simulink model "dynamic_model"  (R2016b)
settings: Solver=ode3  StartTime=0.0  StopTime=inf  FixedStep=0.001  MaxStep=0.004  RelTol=1e-3
undefined symbols (not defined in the file): deg, rad, s
libraries: simulink x6, aerolibconvert2 x3, aerolibobsolete x1, aerolibtransform2 x1, aerolibatmos2 x1, aerolibnav x1, aerolibanimutils x1
settings Model: Creator=ADAM  LastModifiedBy=consti
settings SolverCC: ExtrapolationOrder=1
settings DataIOCC: MaxDataPoints=1  SaveFormat=Structure  SignalLoggingSaveFormat=ModelDataLogs  SaveOutput=off  SignalLogging=off  DSMLogging=off  SaveTime=off  OutputSaveName=model_out  SignalLoggingName=model_out
settings OptimizationCC: ExpressionDepthLimit=2147483647  LifeSpan=inf  SimCompilerOptimization=on
settings DebuggingCC: UnderspecifiedInitializationDetection=Classic  MergeDetectMultiDrivingBlocksExec=none  SolverPrmCheckMsg=warning  InheritedTsInSrcMsg=none  MultiTaskDSMMsg=warning  MultiTaskCondExecSysMsg=none  UnconnectedInputMsg=none  UnconnectedOutputMsg=none  UnconnectedLineMsg=none  StateNameClashWarn=warning  SFUnexpectedBacktrackingDiag=warning  SFNoUnconditionalDefaultTransitionDiag=warning  SFExecutionAtInitializationDiag=none
settings HardwareCC: ProdBitPerPointer=32  ProdBitPerSizeT=32  ProdBitPerPtrDiffT=32  ProdLargestAtomicFloat=None  ProdWordSize=32  ProdHWDeviceType=Generic->32-bit x86 compatible
settings ModelReferenceCC: ModelReferenceNumInstancesAllowed=Single  PropagateSignalLabelsOutOfModel=off
settings CodeAppCC: MaxIdLength=95
settings GRTTargetCC: TargetLangStandard=C89/C90 (ANSI)  GeneratePreprocessorConditionals=Disable all
settings ConfigComp: CovMetricSettings=dw  CovHtmlReporting=on  CovSaveCumulativeToWorkspaceVar=on  CovSaveSingleToWorkspaceVar=on  CovExternalEMLEnable=off  CovSFcnEnable=off

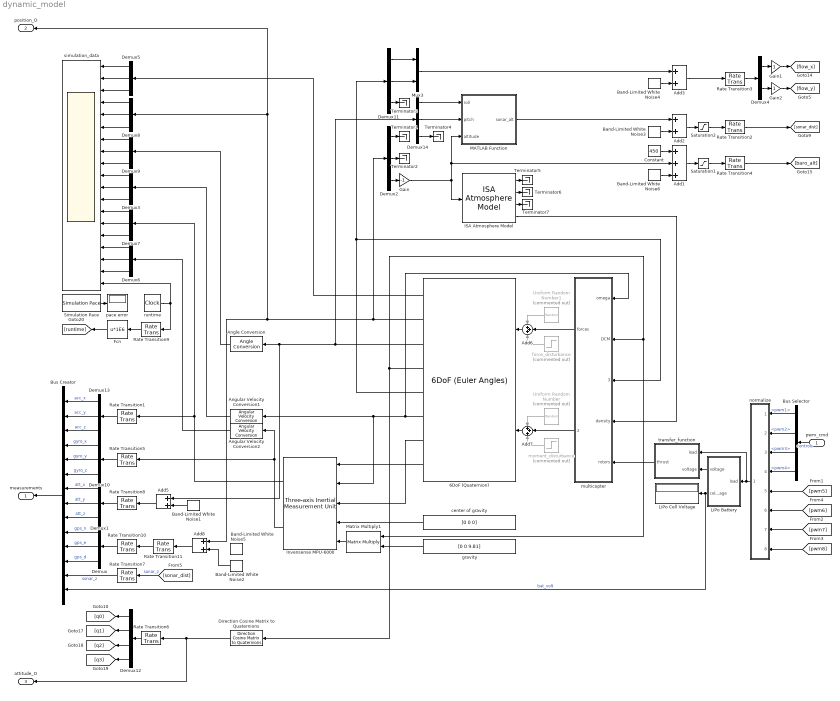
== system dynamic_model ==
  pwm_cmd : Inport  OutDataTypeStr=Bus: Motor_Bus  SampleTime=[0.0040000000000000001,0]
  6DoF (Quaternion) : aerolibobsolete/6DoF (Euler Angles)  units=Metric (MKS)  mtype=Fixed  rep=Quaternion  xme_0=[0 0 -1]  Vm_0=[0 0 0]  eul_0=[0 0 pi]  pm_0=[0 0 0]  mass_0=0.26  mass_e=0  mass_f=0  inertia=[0.00080, 0, 0; 0, 0.00065, 0; 0, 0, 0.0014]  inertia_e=eye(3)  inertia_f=eye(3)  k_quat=1.0
  Add1 : Sum  Inputs=+++
  Add{2..3,5,8} (4 alike) : Sum
  Add6 : Sum  Inputs=+++
  Add7 : Sum  Inputs=+++
  Angle Conversion : aerolibconvert2/Angle Conversion  IU=rad  OU=deg
  Angular Velocity Conversion1 : aerolibconvert2/Angular Velocity Conversion  IU=rad/s  OU=deg/s
  Angular Velocity Conversion2 : aerolibconvert2/Angular Velocity Conversion  IU=rad/s  OU=deg/s
  Band-Limited White Noise1 : simulink/Sources/Band-Limited White Noise  Cov=0.00000000015  Ts=0.004  seed=[243584]
  Band-Limited White Noise2 : simulink/Sources/Band-Limited White Noise  Cov=[0.00003 0.00003 0.00004]  Ts=0.004  seed=[243584 32434 2584]
  Band-Limited White Noise3 : simulink/Sources/Band-Limited White Noise  Cov=0.000005  Ts=0.1  seed=[31841]
  Band-Limited White Noise4 : simulink/Sources/Band-Limited White Noise  Cov=0.000000003  Ts=0.004  seed=[25481]
  Band-Limited White Noise5 : simulink/Sources/Band-Limited White Noise  Cov=[0.0000 0 0.0000]  Ts=0.004  seed=[243584 32434 2584]
  Band-Limited White Noise6 : simulink/Sources/Band-Limited White Noise  Cov=0.0005  Ts=0.008  seed=[79648]
  Bus Creator : BusCreator  Inputs=14
  Bus Selector : BusSelector  OutputSignals=pwm1,pwm2,pwm3,pwm4
  Constant : Constant  Value=450
  Demux{,1..3,5..11,13..14} (13 alike) : Demux  Outputs=3
  Demux12 : Demux
  Demux4 : Demux  Outputs=2
  Direction Cosine Matrix to Quaternions : aerolibtransform2/Direction Cosine Matrix  to Quaternions
  Fcn : Fcn  Expr=u*1E6
      mask Display: fprintf('uS');
  Gain : Gain  Gain=-1
  Gain1 : Gain
  Gain2 : Gain
  ISA Atmosphere Model : aerolibatmos2/ISA Atmosphere Model  custom=on  g=9.80665  gamma=1.4  R=287.0531  L=0.0065  h_trop=11000  h_strat=20000  rho0=1.225  P0=101325  T0=288.15  h0=-10
  Invensense MPU-6000 : aerolibnav/Three-axis Inertial Measurement Unit  units=Metric (MKS)  imu=[0 0 0]  i_Ts=0.004  dtype_a=off  w_a=190  z_a=0.707  a_sf_cc=[0.98 0 0; 0 0.98 0; 0 0 0.98]  a_bias=[0 0 0]  a_sat="[-19.62  -19.62  -19.62 19.62 19.62 19.62]"  dtype_g=off  w_g=190  z_g=0.707  g_sf_cc=[.98 0 0; 0 .98 0; 0 0 .98]  g_bias=[0 0 0]  g_sens=[0 0 0]  g_sat="[-4.36  -4.36  -4.36 4.36 4.36 4.36]"  i_rand=on  i_seeds=[348631 366719 978432 189621 128794 214632]  i_pow=[0.0000005 0.0000005 0.0000005 0.000000002 0.000000002 0.000000002]
  LiPo Battery : MATLAB Function  TreatAsAtomicUnit=on  SystemSampleTime=0.004
  LiPo Cell Voltage : Display
  MATLAB Function : MATLAB Function  TreatAsAtomicUnit=on
  Matrix Multiply1 : Product  Multiplication=Matrix(*)
  Mux3 : Mux  Inputs=2
  Rate Transition{1,3,5..10} (8 alike) : RateTransition  OutPortSampleTime=0.004
  Rate Transition11 : RateTransition  OutPortSampleTime=0.2
  Rate Transition2 : RateTransition  OutPortSampleTime=0.1
  Rate Transition4 : RateTransition  OutPortSampleTime=0.008
  Saturation1 : Saturate  UpperLimit=inf  LowerLimit=0
  Saturation2 : Saturate  UpperLimit=5  LowerLimit=0.3
  Simulation Pace : aerolibanimutils/Simulation Pace  SimulationPace=1  SleepMode=MATLAB Thread  OutputPaceError=on  SampleTime=0.004
      settings: AttributesFormatString=%<SimulationPace> sec/sec
  Terminator{1..7} (7 alike) : Terminator
  Uniform Random Number : UniformRandomNumber  Commented=on  Minimum=[-0.0005 -0.0005 -0.0001]  Maximum=[0.0005 0.0005 0.0001]  SampleTime=5
  Uniform Random Number1 : UniformRandomNumber  Commented=on  Minimum=[-0.01 -0.01 -0.1]  Maximum=[0.01 0.01 0.1]  SampleTime=5
  center of gravity : Constant  Value=[0 0 0]
  force_disturbance : Step  Commented=on  Time=5  Before=[0 0 0]  After=[0 0 0]
  gravity : Constant  Value=[0 0 9.81]
  moment_disturbance : Step  Commented=on  Time=5  Before=[0 0 0]  After=[0 0 0]
  multicopter : MATLAB Function  TreatAsAtomicUnit=on
  normalize : Subsystem
      mask Display:
      | port_label('input', 1, 'pwm1');
      | port_label('input', 2, 'pwm2');
      | port_label('input', 3, 'pwm3');
      | port_label('input', 4, 'pwm4');
      | port_label('input', 5, 'pwm5');
      | port_label('input', 6, 'pwm6');
      | port_label('input', 7, 'pwm7');
      | port_label('input', 8, 'pwm8');
  pace error : Display
  runtime : DigitalClock  SampleTime=0.00100000000000000002
  simulation_data : Scope  NumInputPorts=19
  transfer_function : Subsystem
      mask Display: fprintf('Brushless Motors')
  measurements : Outport  OutDataTypeStr=Bus: Sensor_Bus  SampleTime=[0.0040000000000000001,0]
  position_O : Outport  Port=2  OutDataTypeStr=double  PortDimensions=3  SampleTime=0
  attitude_O : Outport  Port=3  OutDataTypeStr=double  PortDimensions=4  SampleTime=0
  wires:
  6DoF (Quaternion)/7 -> Invensense MPU-6000/3
  Demux1/1 -> Bus Creator/7  "att_x"
  6DoF (Quaternion)/3 -> Add5/1, Angle Conversion/1, Demux14/1
  6DoF (Quaternion)/8 -> Invensense MPU-6000/1
  6DoF (Quaternion)/5 -> multicopter/3(velocity), Demux11/1
  Demux9/1 -> simulation_data/7
  Demux9/2 -> simulation_data/8
  Demux3/1 -> simulation_data/10
  Demux3/2 -> simulation_data/11
  Demux3/3 -> simulation_data/12
  Demux7/1 -> simulation_data/13
  Demux7/2 -> simulation_data/14
  Demux7/3 -> simulation_data/15
  Demux/1 -> Bus Creator/10  "gps_n"
  Demux/2 -> Bus Creator/11  "gps_e"
  Demux/3 -> Bus Creator/12  "gps_d"
  Demux1/2 -> Bus Creator/8  "att_y"
  Demux5/1 -> simulation_data/1
  Demux5/2 -> simulation_data/2
  Demux5/3 -> simulation_data/3
  Demux8/1 -> simulation_data/4
  Demux8/2 -> simulation_data/5
  Demux8/3 -> simulation_data/6
  6DoF (Quaternion)/6 -> Angular Velocity Conversion1/1, Invensense MPU-6000/2, multicopter/1(omega)
  Demux9/3 -> simulation_data/9
  Demux6/1 -> simulation_data/16
  Demux6/2 -> simulation_data/17
  Demux6/3 -> simulation_data/18
  Angular Velocity Conversion2/1 -> Demux6/1
  Demux10/1 -> Bus Creator/4  "gyro_x"
  Demux10/2 -> Bus Creator/5  "gyro_y"
  Demux10/3 -> Bus Creator/6  "gyro_z"
  6DoF (Quaternion)/4 -> Direction Cosine Matrix to Quaternions/1, multicopter/2(DCM), Matrix Multiply1/1
  Simulation Pace/1 -> pace error/1
  6DoF (Quaternion)/1 -> Demux5/1
  6DoF (Quaternion)/2 -> Add8/1, position_O/1, Demux8/1, Demux2/1
  Angle Conversion/1 -> Demux9/1
  Angular Velocity Conversion1/1 -> Demux3/1
  Invensense MPU-6000/1 -> Demux7/1, Rate Transition1/1
  Invensense MPU-6000/2 -> Angular Velocity Conversion2/1, Rate Transition5/1
  runtime/1 -> Rate Transition9/1, simulation_data/19
  Rate Transition6/1 -> Demux12/1
  Demux12/4 -> [q3]
  Demux12/3 -> [q2]
  Demux12/2 -> [q1]
  Demux12/1 -> [q0]
  Fcn/1 -> [runtime]
  Rate Transition9/1 -> Fcn/1
  normalize/1(normalized_signals) -> LiPo Battery/1(load), transfer_function/1(load)
  LiPo Battery/1(voltage) -> transfer_function/2(voltage)
  transfer_function/1(thrust) -> multicopter/5(rotors)
  LiPo Battery/2(cell_voltage) -> Bus Creator/14, LiPo Cell Voltage/1  "bat_volt"
  Demux13/2 -> Bus Creator/2  "acc_y"
  Demux13/3 -> Bus Creator/3  "acc_z"
  Band-Limited White Noise1/1 -> Add5/2
  Add6/1 -> 6DoF (Quaternion)/1
  Add7/1 -> 6DoF (Quaternion)/2
  center of gravity/1 -> Invensense MPU-6000/4
  gravity/1 -> Matrix Multiply1/2
  Matrix Multiply1/1 -> Invensense MPU-6000/5
  moment_disturbance/1 -> Add7/3
  multicopter/2(moments) -> Add7/2
  force_disturbance/1 -> Add6/3
  multicopter/1(forces) -> Add6/2
  Uniform Random Number1/1 -> Add6/1
  Uniform Random Number/1 -> Add7/1
  Rate Transition3/1 -> Demux4/1
  Add3/1 -> Rate Transition3/1
  Demux2/3 -> Gain/1
  Gain/1 -> Add1/2, MATLAB Function/3(altitude), ISA Atmosphere Model/1
  Demux2/2 -> Terminator2/1
  Demux2/1 -> Terminator1/1
  Demux11/1 -> Mux3/1
  Demux11/2 -> Mux3/2
  Demux11/3 -> Terminator3/1
  Rate Transition2/1 -> [sonar_dist]
  Rate Transition4/1 -> [baro_alt]
  Saturation1/1 -> Rate Transition4/1
  Saturation2/1 -> Rate Transition2/1
  Add1/1 -> Saturation1/1
  MATLAB Function/1(sonar_alt) -> Add2/1
  Band-Limited White Noise3/1 -> Add2/2
  Add2/1 -> Saturation2/1
  Band-Limited White Noise4/1 -> Add3/2
  Band-Limited White Noise6/1 -> Add1/3
  Constant/1 -> Add1/1
  Mux3/1 -> Add3/1
  Demux4/2 -> Gain2/1
  Demux4/1 -> Gain1/1
  Gain1/1 -> [flow_x]
  Gain2/1 -> [flow_y]
  Demux14/2 -> MATLAB Function/2(pitch)
  Demux14/1 -> MATLAB Function/1(roll)
  Demux14/3 -> Terminator4/1
  ISA Atmosphere Model/3 -> Terminator7/1
  ISA Atmosphere Model/2 -> Terminator6/1
  ISA Atmosphere Model/1 -> Terminator5/1
  ISA Atmosphere Model/4 -> multicopter/4(density)
  Direction Cosine Matrix to Quaternions/1 -> attitude_O/1, Rate Transition6/1
  pwm_cmd/1 -> Bus Selector/1  "controls"
  Bus Selector/1 -> normalize/1(pwm1)  "<pwm1>"
  Bus Selector/2 -> normalize/2(pwm2)  "<pwm2>"
  Bus Selector/3 -> normalize/3(pwm3)  "<pwm3>"
  Bus Selector/4 -> normalize/4(pwm4)  "<pwm4>"
  [pwm5] -> normalize/5(pwm5)
  [pwm6] -> normalize/6(pwm6)
  [pwm7] -> normalize/7(pwm7)
  [pwm8] -> normalize/8(pwm8)
  Bus Creator/1 -> measurements/1
  Demux1/3 -> Bus Creator/9  "att_z"
  Rate Transition10/1 -> Demux/1
  Rate Transition7/1 -> Bus Creator/13  "sonar_z"
  Add8/1 -> Rate Transition11/1
  Rate Transition11/1 -> Rate Transition10/1
  Demux13/1 -> Bus Creator/1  "acc_x"
  Add5/1 -> Rate Transition8/1
  Rate Transition5/1 -> Demux10/1
  Rate Transition1/1 -> Demux13/1
  Rate Transition8/1 -> Demux1/1
  [sonar_dist] -> Rate Transition7/1  "sonar_z"
  Band-Limited White Noise2/1 -> Add8/2

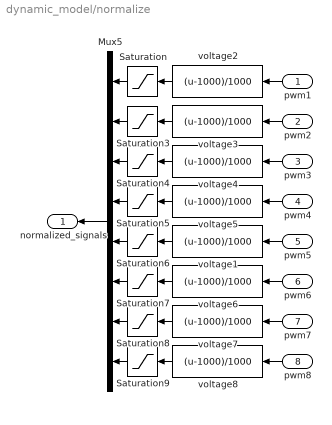
== system dynamic_model/normalize ==
  pwm1 : Inport
  pwm2 : Inport  Port=2
  pwm3 : Inport  Port=3
  pwm4 : Inport  Port=4
  pwm5 : Inport  Port=5
  pwm6 : Inport  Port=6
  pwm7 : Inport  Port=7
  pwm8 : Inport  Port=8
  Mux5 : Mux  Inputs=8
  Saturation{,3..9} (8 alike) : Saturate  UpperLimit=1  LowerLimit=0
  voltage{1..8} (8 alike) : Fcn  Expr=(u-1000)/1000
  normalized_signals : Outport
  wires:
  voltage3/1 -> Saturation3/1
  Saturation3/1 -> Mux5/2
  Saturation/1 -> Mux5/1
  Saturation6/1 -> Mux5/5
  voltage1/1 -> Saturation6/1
  pwm2/1 -> voltage3/1
  pwm5/1 -> voltage1/1
  pwm4/1 -> voltage5/1
  pwm8/1 -> voltage8/1
  pwm6/1 -> voltage6/1
  pwm7/1 -> voltage7/1
  Saturation4/1 -> Mux5/3
  voltage4/1 -> Saturation4/1
  pwm1/1 -> voltage2/1
  Mux5/1 -> normalized_signals/1
  pwm3/1 -> voltage4/1
  Saturation9/1 -> Mux5/8
  voltage8/1 -> Saturation9/1
  Saturation8/1 -> Mux5/7
  voltage7/1 -> Saturation8/1
  voltage2/1 -> Saturation/1
  voltage5/1 -> Saturation5/1
  voltage6/1 -> Saturation7/1
  Saturation7/1 -> Mux5/6
  Saturation5/1 -> Mux5/4

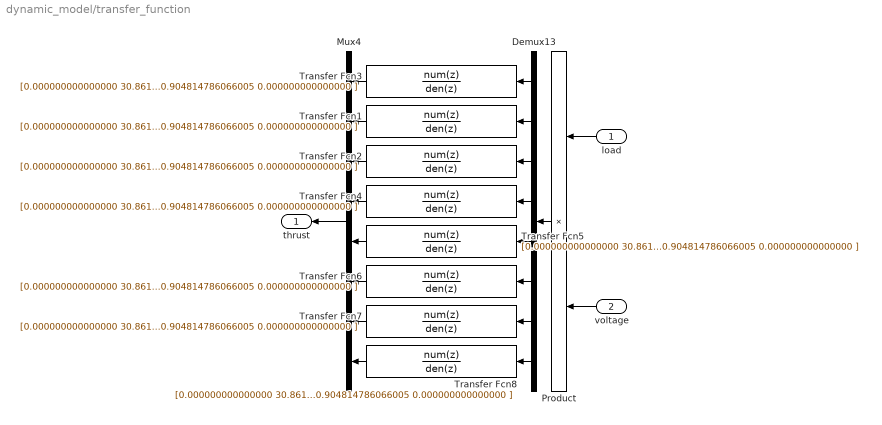
== system dynamic_model/transfer_function ==
  load : Inport  PortDimensions=[8]
  voltage : Inport  Port=2  PortDimensions=[8]
  Demux13 : Demux  Outputs=8
  Mux4 : Mux  Inputs=8
  Product : Product
  Transfer Fcn1 : DiscreteTransferFcn  Numerator=[0.000000000000000 30.861623144040156 0.073571384506755 ]  Denominator=[1.000000000000000 -0.904814786066005 0.000000000000000 ]  SampleTime=0.00100000000000000002  mask(DiscretizedDiscreteTransferFcn){}
      mask init:
      | %zoh
  Transfer Fcn2 : DiscreteTransferFcn  Numerator=[0.000000000000000 30.861623144040156 0.073571384506755 ]  Denominator=[1.000000000000000 -0.904814786066005 0.000000000000000 ]  SampleTime=0.00100000000000000002  mask(DiscretizedDiscreteTransferFcn){}
      mask init:
      | %zoh
  Transfer Fcn3 : DiscreteTransferFcn  Numerator=[0.000000000000000 30.861623144040156 0.073571384506755 ]  Denominator=[1.000000000000000 -0.904814786066005 0.000000000000000 ]  SampleTime=0.00100000000000000002  mask(DiscretizedDiscreteTransferFcn){}
      mask init:
      | %zoh
  Transfer Fcn4 : DiscreteTransferFcn  Numerator=[0.000000000000000 30.861623144040156 0.073571384506755 ]  Denominator=[1.000000000000000 -0.904814786066005 0.000000000000000 ]  SampleTime=0.00100000000000000002  mask(DiscretizedDiscreteTransferFcn){}
      mask init:
      | %zoh
  Transfer Fcn5 : DiscreteTransferFcn  Numerator=[0.000000000000000 30.861623144040156 0.073571384506755 ]  Denominator=[1.000000000000000 -0.904814786066005 0.000000000000000 ]  SampleTime=0.00100000000000000002  mask(DiscretizedDiscreteTransferFcn){}
      mask init:
      | %zoh
  Transfer Fcn6 : DiscreteTransferFcn  Numerator=[0.000000000000000 30.861623144040156 0.073571384506755 ]  Denominator=[1.000000000000000 -0.904814786066005 0.000000000000000 ]  SampleTime=0.00100000000000000002  mask(DiscretizedDiscreteTransferFcn){}
      mask init:
      | %zoh
  Transfer Fcn7 : DiscreteTransferFcn  Numerator=[0.000000000000000 30.861623144040156 0.073571384506755 ]  Denominator=[1.000000000000000 -0.904814786066005 0.000000000000000 ]  SampleTime=0.00100000000000000002  mask(DiscretizedDiscreteTransferFcn){}
      mask init:
      | %zoh
  Transfer Fcn8 : DiscreteTransferFcn  Numerator=[0.000000000000000 30.861623144040156 0.073571384506755 ]  Denominator=[1.000000000000000 -0.904814786066005 0.000000000000000 ]  SampleTime=0.00100000000000000002  mask(DiscretizedDiscreteTransferFcn){}
      mask init:
      | %zoh
  thrust : Outport
  wires:
  load/1 -> Product/1
  Mux4/1 -> thrust/1
  Product/1 -> Demux13/1
  voltage/1 -> Product/2
  Demux13/4 -> Transfer Fcn4/1
  Demux13/3 -> Transfer Fcn2/1
  Demux13/2 -> Transfer Fcn1/1
  Demux13/1 -> Transfer Fcn3/1
  Transfer Fcn6/1 -> Mux4/6
  Transfer Fcn3/1 -> Mux4/1
  Demux13/5 -> Transfer Fcn5/1
  Transfer Fcn5/1 -> Mux4/5
  Transfer Fcn7/1 -> Mux4/7
  Demux13/7 -> Transfer Fcn7/1
  Transfer Fcn1/1 -> Mux4/2
  Transfer Fcn8/1 -> Mux4/8
  Demux13/8 -> Transfer Fcn8/1
  Transfer Fcn2/1 -> Mux4/3
  Transfer Fcn4/1 -> Mux4/4
  Demux13/6 -> Transfer Fcn6/1

== matlab function dynamic_model/MATLAB Function ==
  data: roll input; pitch input; altitude input; sonar_alt output
function sonar_alt = ultrasonic(roll, pitch, altitude)
if altitude > 0
    sonar_alt = sqrt(altitude^2 + (sqrt((altitude*tan(roll))^2 + (altitude*tan(pitch))^2))^2);
else
    sonar_alt = 0;
end

== matlab function dynamic_model/LiPo Battery ==
  data: load input; voltage output; cell_voltage output
function [voltage, cell_voltage]= LiPo(load)

%================================Constants=================================

delta_t = 0.004;
max_current = 5.500;                % maximum current per motor             (A)
aux_current = 0.100;                % current of auxillary components       (A)        
capacity = 1.000;                   % LiPo current capacity                 (Ah)                                 
cells = 2;                          % LiPo cell count

%==========================================================================

persistent discharge;

if isempty(discharge)
    discharge = 0;
end

current = sum(max_current .* load.^2) + aux_current;
discharge = current * (delta_t / 3600) + discharge;

discharge_capacity = discharge / capacity;

if (0 < discharge_capacity) && (discharge_capacity <=0.20)
    cell_voltage = -14.029*discharge_capacity^3 + 16.975*discharge_capacity^2 - 5.3339*discharge_capacity + 4.2;
elseif (0.20 < discharge_capacity) && (discharge_capacity < 0.70)
    cell_voltage = -0.2*discharge_capacity + 3.74;
else
    cell_voltage = -48*discharge_capacity^3 + 89.6*discharge_capacity^2 - 55.08*discharge_capacity + 14.716;
end

if cell_voltage < (5 / cells)
    cell_voltage = 0;
end

supply_voltage = cells * cell_voltage;
voltage = supply_voltage .* load;

%==========================================================================

== matlab function dynamic_model/multicopter ==
  data: omega input; DCM input; velocity input; density input; rotors input; forces output; moments output
function [forces, moments] = multicopter(omega, DCM, velocity, density, rotors)

%================================Constants=================================

coefficient_drag = 15;              % coefficient of drag
rotor_inertia = 0.0000025;          % rotor inertia                         (kg m^2)
prop_diameter = 0.1397;             % diameter of the propellor             (meters)                                 
aircraft_mass = 0.26;               % aircraft mass                         (kg)                                        
aircraft_diameter = 0.25;           % motor to motor distance               (meters)                                      

%==============================Actuator Mixer==============================

% [x(roll), y(pitch), z(yaw)]


MIX = [  1   1  -1   ;      % QUAD [X]
        -1   1   1   ;
        -1  -1  -1   ;
         1  -1   1   ;
         0   0   0   ;
         0   0   0   ;
         0   0   0   ;
         0   0   0   ];

% MIX = [  0   1  -1   ;      % QUAD [+]
%         -1   0   1   ;
%          0  -1  -1   ;
%          1   0   1   ;
%          0   0   0   ;
%          0   0   0   ;
%          0   0   0   ;
%          0   0   0   ];

% MIX = [  1   1  -1   ;      % HEX [X]
%         -1   1   1   ;
%         -1   0  -1   ;
%         -1  -1   1   ;
%          1  -1  -1   ;
%          1   0   1   ;
%          0   0   0   ;
%          0   0   0   ];

%==================================Forces================================== 

a = [   aircraft_diameter^2 / 10                        ;...                % body cross sectional area (X)
        aircraft_diameter^2 / 10                        ;...                % body cross sectional area (Y)
        sum(abs(MIX(:, 3))) * pi/4 * prop_diameter^2    ];                  % body cross sectional area (Z)
    
gravity = aircraft_mass .* (DCM * [0; 0; 9.81]);                            % gravitational force
drag = -velocity .* coefficient_drag .* density .* a;                       % drag force

%--------------------------------Thrust Model------------------------------
thrust = abs(MIX(:, 3)) .* (1*1E-3) .* rotors;                              % rotor thrust <==     
%--------------------------------------------------------------------------

forces = gravity + drag;
forces(3) = forces(3) - sum(thrust);

%==================================Moments=================================

mx = thrust .* MIX(:,1) .* (aircraft_diameter / 2)*sind(45);                % x moment
my = thrust .* MIX(:,2) .* (aircraft_diameter / 2)*sind(45);                % y moment

momentum_x = sum(abs(MIX(:, 3)) .* rotor_inertia .* rotors) * omega(1);     % x rotor momentum
momentum_y = sum(abs(MIX(:, 3)) .* rotor_inertia .* rotors) * omega(2);     % y rotor momentum
momentum_z = sum(MIX(:, 3) .* rotor_inertia .* rotors) * omega(3);          % z rotor momentum

%--------------------------------Torque Model------------------------------
mz = MIX(:,3) .* (1.7E-5) .* rotors;                                        % rotor torque <==
%--------------------------------------------------------------------------

moments = [sum(mx); sum(my); sum(mz)] - [momentum_x; momentum_y; momentum_z];

%==========================================================================
